simulink model "pendcart"  (Simulink 8.9)
settings: Solver=ode45  StartTime=0.0  StopTime=tsim  RelTol=1e-3  EnableMultiTasking=on
values from neighbouring files (symbols this model uses):
  b = 0.01    [pendcartsim.m]
  c = 0.05    [pendcartsim.m]
  g = 9.82    [pendcartsim.m]
  K1 = -119.0071    [pendcartsim.m]
  K2 = 0.0402    [pendcartsim.m]
  l = 0.5    [pendcartsim.m]
  M = 1    [pendcartsim.m]
  m = 0.5    [pendcartsim.m]
  p = 5.4277    [pendcartsim.m]
  p1 = 25.4277    [pendcartsim.m]
  theta0 = 5*pi/180    (= 0.0872664625997)    [pendcartsim.m]
  Wheel_Radius = 0.035    [pendcartsim.m]
undefined symbols (not defined in the file or in its folder): DiscIntNeverNeededParam, sigbuilder_block, Ts
libraries: powerlib x7
settings Model: Creator=Chris  LastModifiedBy=Administrator
settings OptimizationCC: ExpressionDepthLimit=2147483647  InitFltsAndDblsToZero=on
settings DebuggingCC: AlgebraicLoopMsg=none  SaveWithParameterizedLinksMsg=none
settings GRTTargetCC: TargetFcnLib=ansi_tfl_tmw.mat

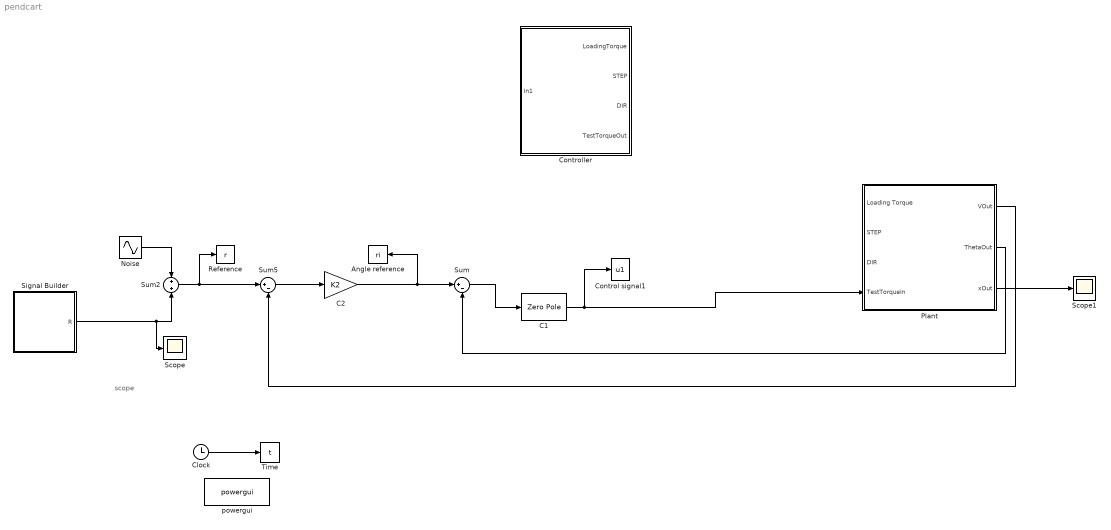
== system pendcart ==
  note: scope
  Angle reference : ToWorkspace  VariableName=ri  SampleTime=-1
  C1 : ZeroPole  Zeros=[-p]  Poles=[-p1]  Gain=[K1]
  C2 : Gain  Gain=K2
  Clock : Clock
  Control signal1 : ToWorkspace  VariableName=u1  SampleTime=-1
  Controller : Subsystem
  "Noise " : Sin  Amplitude=0.01  Frequency=3  SampleTime=0
  Plant : Subsystem
  Reference : ToWorkspace  VariableName=r  SampleTime=-1
  Scope : Scope
  Scope1 : Scope
  Signal Builder : Subsystem  Tag=STV Subsys  LoadFcn=sigbuilder_block('load',[5.5 23 949 425 ]);  StartFcn=sigbuilder_block('start');  StopFcn=sigbuilder_block('stop');  ClipboardFcn=sigbuilder_block('clipboard');  mask(Sigbuilder block){tuvar=[0:10]}
      mask help: Sigbuilder GUI
      mask init:
      | if ~strcmp(get_param(bdroot(gcbh),'SimulationStatus'),'stopped') tuvar = sigbuilder_block('maskInit'); end
      settings: CopyFcn=sigbuilder_block('copy');  DeleteFcn=sigbuilder_block('delete');  ModelCloseFcn=sigbuilder_block('modelClose');  PreSaveFcn=sigbuilder_block('preSave');  PauseFcn=sigbuilder_block('pause')  ContinueFcn=sigbuilder_block('continue')  NameChangeFcn=sigbuilder_block('namechange');  OpenFcn=sigbuilder_block('open',[5.5 23 949 425 ]);  CloseFcn=sigbuilder_block('close');
      mask Display: plot(0, 0, 100, 100,[2, 2, 32, 32, 2], [68, 8, 8, 68, 68],[32, 2], [38, 38], [32, 19, 2],[53, 60, 44], [32, 17, 17, 2],[16, 16, 31, 31]);txt = getActiveGroup(gcbh);text(2, 100, txt,'verticalAlignment', 'top');
  Sum : Sum  Inputs=|+-
  Sum2 : Sum
  Sum5 : Sum  Inputs=|+-
  Time : ToWorkspace  VariableName=t  SampleTime=-1
  powergui : powerlib/powergui  SimulationMode=Discrete  SampleTime=Ts  frequency=60  Iterations=50  frequencyindice=0  Pbase=100e6  ErrMax=1e-4  UnitsV=kV  UnitsW=MW  buscounter=0  FunctionMessages=off  echomessages=off  EnableUseOfTLC=off  CurrentSourceSwitches=off  DisableSnubberDevices=off  DisableRonSwitches=off  DisableVfSwitches=off  DisplayEquations=off  SolverType=Tustin/Backward Euler (TBE)  Interpol=off  ExternalGateDelay=off  methode=off  Ts=0  x0status=blocks  SPID=off  SwTol=0  HookPort=off  RestoreLinks=warning  ResistiveCurrentMeasurement=off  Frange=[0:2:500]  Ylog=off  Xlog=on  ShowGrid=off  save=off  variable=ZData  structure=0  ZoomFFT=on  StartTime=0.0  cycles=1  DisplayStyle=1  fundamental=60  FreqAxis=off  MaxFrequency=1000  frequencyindicesteady=1  RmsSteady=1  display=off
  wires:
  Clock/1 -> Time/1
  Sum5/1 -> C2/1
  C2/1 -> Angle reference/1, Sum/1
  Sum2/1 -> Sum5/1, Reference/1
  "Noise "/1 -> Sum2/1
  Plant/1(VOut) -> Sum5/2
  Plant/2(ThetaOut) -> Sum/2
  ? -> Plant/3(DIR)
  ? -> Plant/2(STEP)
  ? -> Plant/1(Loading Torque)
  C1/1 -> Control signal1/1, Plant/4(TestTorqueIn)
  Sum/1 -> C1/1
  Signal Builder/1(R) -> Scope/1, Sum2/2
  Plant/3(xOut) -> Scope1/1

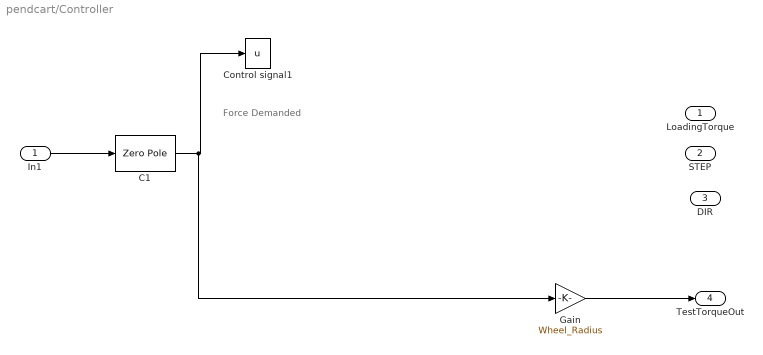
== system pendcart/Controller ==
  note: Force Demanded
  In1 : Inport
  C1 : ZeroPole  Zeros=[-p]  Poles=[-p1]  Gain=[K1]
  Control signal1 : ToWorkspace  VariableName=u  SampleTime=-1
  Gain : Gain  Gain=Wheel_Radius
  LoadingTorque : Outport
  STEP : Outport  Port=2
  DIR : Outport  Port=3
  TestTorqueOut : Outport  Port=4
  wires:
  C1/1 -> Gain/1, Control signal1/1
  In1/1 -> C1/1
  Gain/1 -> TestTorqueOut/1

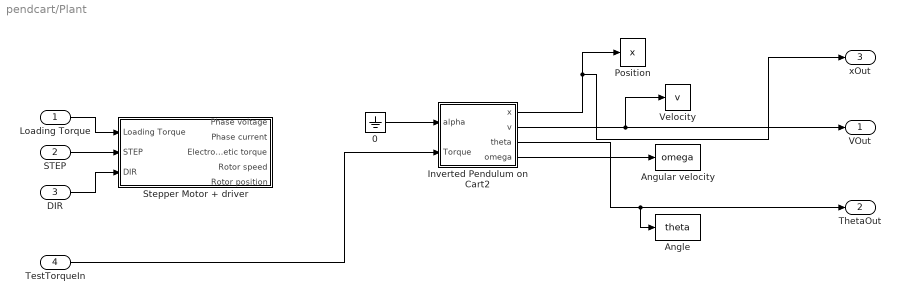
== system pendcart/Plant ==
  Loading Torque : Inport
  STEP : Inport  Port=2
  DIR : Inport  Port=3
  TestTorqueIn : Inport  Port=4
  0 : Ground
  Angle : ToWorkspace  VariableName=theta  SampleTime=-1
  Angular velocity : ToWorkspace  VariableName=omega  SampleTime=-1
  Inverted Pendulum on Cart2 : Subsystem
  Position : ToWorkspace  VariableName=x  SampleTime=-1
  Stepper Motor + driver : Subsystem
  Velocity : ToWorkspace  VariableName=v  SampleTime=-1
  VOut : Outport
  ThetaOut : Outport  Port=2
  xOut : Outport  Port=3
  wires:
  DIR/1 -> Stepper Motor + driver/3(DIR)
  Loading Torque/1 -> Stepper Motor + driver/1(Loading Torque)
  STEP/1 -> Stepper Motor + driver/2(STEP)
  Inverted Pendulum on Cart2/4(omega) -> Angular velocity/1
  Inverted Pendulum on Cart2/1(x) -> xOut/1, Position/1
  Inverted Pendulum on Cart2/3(theta) -> ThetaOut/1, Angle/1
  Inverted Pendulum on Cart2/2(v) -> VOut/1, Velocity/1
  0/1 -> Inverted Pendulum on Cart2/1(alpha)
  TestTorqueIn/1 -> Inverted Pendulum on Cart2/2(Torque)

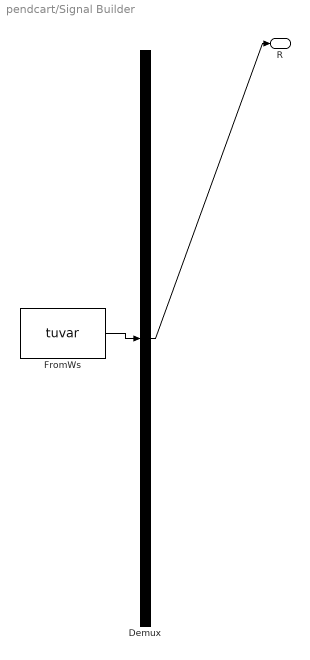
== system pendcart/Signal Builder ==
  Demux : Demux  Tag=STV Demux  Outputs=1
  FromWs : FromWorkspace  Tag=STV FromWs  VariableName=tuvar  SampleTime=0  SigBuilderData=DataTag0  VnvData=DataTag1
      SigBuilderData=|
      | common.afterFinalStr = 'Extrapolate'
      | common.sampleTime = 0
      | dataSet.timeRange = [0 20]
      | dataSet.name = 'Group 1'
      | sbobj.Groups.Name = 'Group 1'
      | sbobj.Groups.Signals.Name = 'R'
      | sbobj.Groups.Signals.XData = [0 8 8 12 12 20]
      | sbobj.Groups.Signals.YData = [0 0.77 1 1 0 0]
      | sbobj.Groups.TimeRange = [0 20]
  R : Outport  Tag=STV Outport
  wires:
  FromWs/1 -> Demux/1
  Demux/1 -> R/1

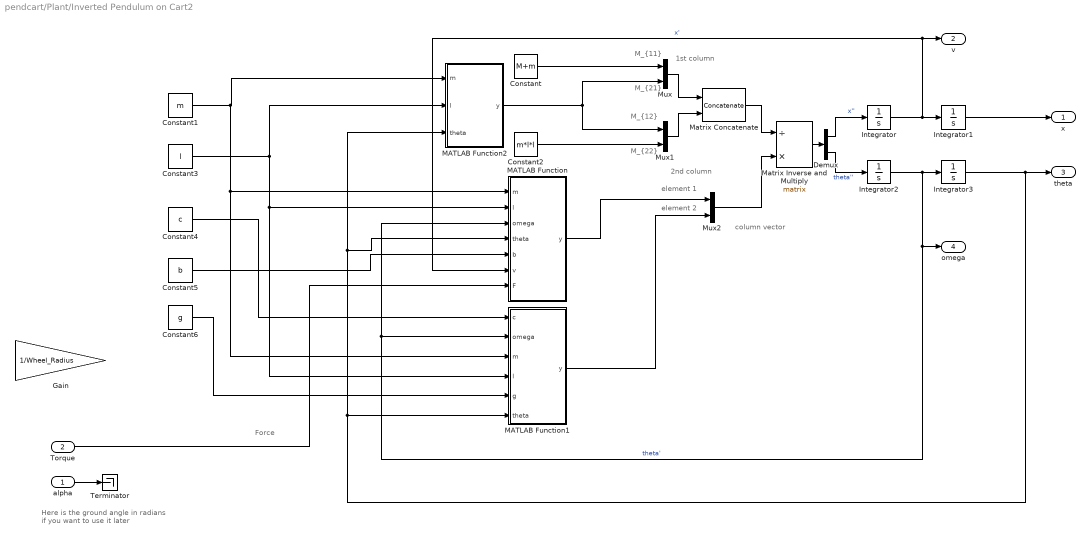
== system pendcart/Plant/Inverted Pendulum on Cart2 ==
  note: Force
  note: 2nd column
  note: M_{21}
  note: 1st column
  note: M_{12}
  note: element 2
  note: Here is the ground angle in
      | radians if you want to use it later
  note: column vector
  note: M_{11}
  note: M_{22}
  note: element 1
  alpha : Inport
  Torque : Inport  Port=2
  Constant : Constant  Value=M+m
  Constant1 : Constant  Value=m
  Constant2 : Constant  Value=m*l*l
  Constant3 : Constant  Value=l
  Constant4 : Constant  Value=c
  Constant5 : Constant  Value=b
  Constant6 : Constant  Value=g
  Demux : Demux  Outputs=2
  Gain : Gain  Gain=1/Wheel_Radius
  Integrator : Integrator
  Integrator1 : Integrator
  Integrator2 : Integrator
  Integrator3 : Integrator  InitialCondition=theta0
  MATLAB Function : MATLAB Function  TreatAsAtomicUnit=on
  MATLAB Function1 : MATLAB Function  TreatAsAtomicUnit=on
  MATLAB Function2 : MATLAB Function  TreatAsAtomicUnit=on
  Matrix Concatenate : Concatenate  Mode=Multidimensional array  ConcatenateDimension=2
  Matrix Inverse and Multiply : Product  Inputs=/*  Multiplication=Matrix(*)
  Mux : Mux  Inputs=2
  Mux1 : Mux  Inputs=2
  Mux2 : Mux  Inputs=2
  Terminator : Terminator
  x : Outport
  v : Outport  Port=2
  theta : Outport  Port=3
  omega : Outport  Port=4
  wires:
  MATLAB Function1/1(y) -> Mux2/2
  Constant1/1 -> MATLAB Function1/3(m), MATLAB Function/1(m), MATLAB Function2/1(m)
  Constant5/1 -> MATLAB Function/5(b)
  Matrix Inverse and Multiply/1 -> Demux/1
  Constant2/1 -> Mux1/2
  Mux2/1 -> Matrix Inverse and Multiply/2
  MATLAB Function/1(y) -> Mux2/1
  Constant4/1 -> MATLAB Function1/1(c)
  Mux1/1 -> Matrix Concatenate/2
  Constant/1 -> Mux/1
  MATLAB Function2/1(y) -> Mux1/1, Mux/2
  Integrator/1 -> Integrator1/1, v/1, MATLAB Function/6(v)  "x'"
  Matrix Concatenate/1 -> Matrix Inverse and Multiply/1
  Integrator1/1 -> x/1
  Demux/2 -> Integrator2/1  "theta''"
  Integrator3/1 -> MATLAB Function/4(theta), MATLAB Function2/3(theta), MATLAB Function1/6(theta), theta/1
  Constant3/1 -> MATLAB Function1/4(l), MATLAB Function/2(l), MATLAB Function2/2(l)
  Mux/1 -> Matrix Concatenate/1
  Integrator2/1 -> Integrator3/1, MATLAB Function/3(omega), MATLAB Function1/2(omega), omega/1  "theta'"
  Constant6/1 -> MATLAB Function1/5(g)
  alpha/1 -> Terminator/1
  Demux/1 -> Integrator/1  "x''"
  Torque/1 -> MATLAB Function/7(F)

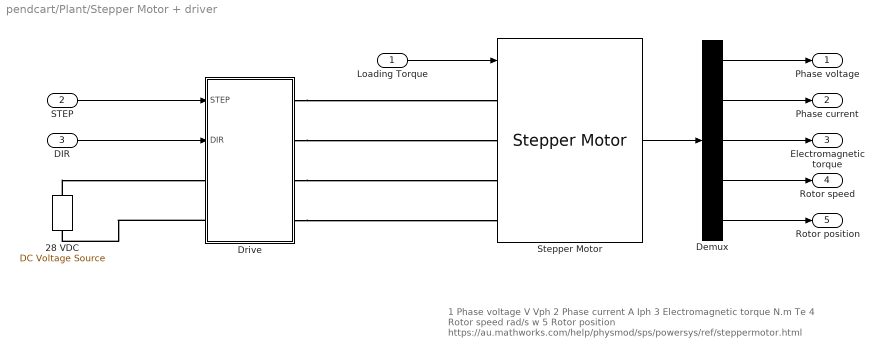
== system pendcart/Plant/Stepper Motor + driver ==
  note: 1
      | Phase voltage
      | V
      | Vph
      |
      | 2
      | Phase current
      | A
      | Iph
      |
      | 3
      | Electromagnetic torque
      | N.m
      | Te
      |
      | 4
      | Rotor speed
      | rad/s
      | w
      |
      | 5
      | Rotor position
      |
      | https://au.mathworks.com/help/physmod/sps/powersys/ref/steppermotor.html
  Loading Torque : Inport
  STEP : Inport  Port=2
  DIR : Inport  Port=3
  28 VDC : powerlib/Electrical Sources/DC Voltage Source  Amplitude=28  Measurements=None
  Demux : Demux  Outputs=5
  Drive : Subsystem  mask{Iref=2, step=500, Ts=Ts}
      mask prompts: Iref "Phase current (A)"; step "Stepping rate (step/s)"; Ts "Sampling time (s)"
      mask init:
      | Nstep=round(1/step/Ts);
  Stepper Motor : powerlib/Machines/Stepper Motor  MotorType=Permanent-magnet / Hybrid  NumberOfPhases_1=2  NumberOfPhases_2=3  PresetModel_1=<empty>  PresetModel_2=<empty>  L=10e-3  Lmax=10e-3  Lmin=2e-3  R=1.2  Step_angle=30  Psim=0.04  Tdm=0.02  J=1e-4/5  B=1e-3  w0=0  pos0=0  TsPowergui=0  TsBlock=-1
      settings: SourceProductName=Simscape Power Systems  SourceProductBaseCode=PS
  Phase voltage : Outport
  Phase current : Outport  Port=2
  Electromagnetic torque : Outport  Port=3
  Rotor speed : Outport  Port=4
  Rotor position : Outport  Port=5
  wires:
  Demux/2 -> Phase current/1
  Loading Torque/1 -> Stepper Motor/1
  Demux/3 -> Electromagnetic torque/1
  Demux/1 -> Phase voltage/1
  Demux/4 -> Rotor speed/1
  Stepper Motor/1 -> Demux/1
  Demux/5 -> Rotor position/1
  DIR/1 -> Drive/2(DIR)
  STEP/1 -> Drive/1(STEP)
  connections:
  Drive/RConn3 -- Stepper Motor/LConn3
  Drive/LConn2 -- 28 VDC/LConn1
  28 VDC/RConn1 -- Drive/LConn1
  Drive/RConn1 -- Stepper Motor/LConn1
  Drive/RConn2 -- Stepper Motor/LConn2
  Drive/RConn4 -- Stepper Motor/LConn4

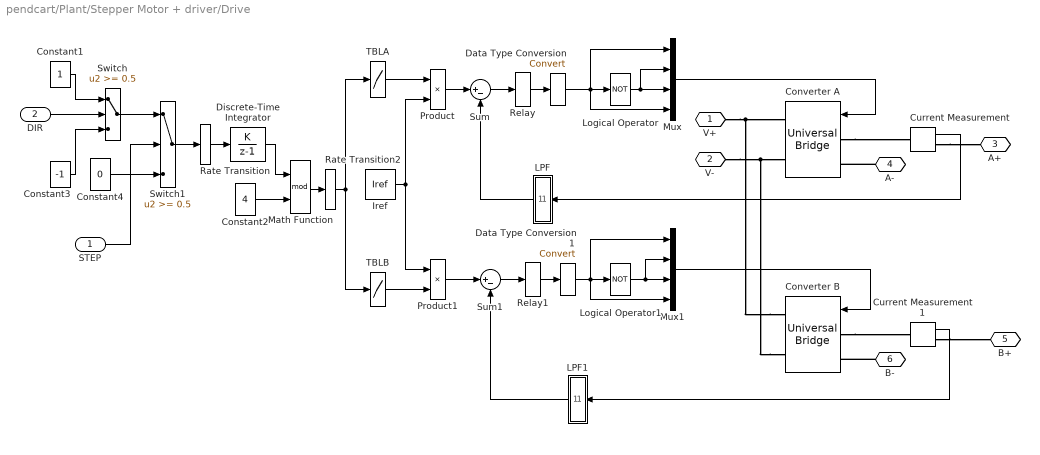
== system pendcart/Plant/Stepper Motor + driver/Drive ==
  STEP : Inport
  DIR : Inport  Port=2
  Constant1 : Constant  SampleTime=Ts
  Constant2 : Constant  Value=4  SampleTime=Nstep*Ts
  Constant3 : Constant  Value=-1  SampleTime=Ts
  Constant4 : Constant  Value=0  SampleTime=Ts
  Converter A : powerlib/Power Electronics/Universal Bridge  Arms=2  SnubberResistance=10000  SnubberCapacitance=inf  Device=MOSFET / Diodes  Ron=1e-3*10  Lon=0  ForwardVoltages="[  0  0  ]"  ForwardVoltage=0  GTOparameters=[ 10e-6 , 20e-6 ]  IGBTparameters=[ 0.5e-6 , 0.5e-6 ]  Measurements=None  Measurements_2=None  converterType=Rectifier
  Converter B : powerlib/Power Electronics/Universal Bridge  Arms=2  SnubberResistance=10000  SnubberCapacitance=inf  Device=MOSFET / Diodes  Ron=1e-3*10  Lon=0  ForwardVoltages="[  0  0  ]"  ForwardVoltage=0  GTOparameters=[ 10e-6 , 20e-6 ]  IGBTparameters=[ 0.5e-6 , 0.5e-6 ]  Measurements=None  Measurements_2=None  converterType=Rectifier
  Current Measurement : powerlib/Measurements/Current Measurement  PhasorSimulation=off  OutputType=Complex  PSBequivalent=0
  Current Measurement1 : powerlib/Measurements/Current Measurement  PhasorSimulation=off  OutputType=Complex  PSBequivalent=0
  Data Type Conversion : DataTypeConversion
  Data Type Conversion1 : DataTypeConversion
  Discrete-Time Integrator : DiscreteIntegrator  IntegratorMethod=Accumulation: Forward Euler  SampleTime=Nstep*Ts  ICPrevOutput=DiscIntNeverNeededParam  ICPrevScaledInput=DiscIntNeverNeededParam
  Iref : Constant  Value=Iref  SampleTime=Ts
  LPF : Subsystem  mask{fc=10000, Ts=Ts}
      mask prompts: fc "Cut-off frequency (Hz)"; Ts "Sampling time (s)"
      mask init:
      | % fa=tf(1,[1/2/pi/fc 1]);
      | % fn=c2d(fa,Ts);
      | % [NN,DD]=tfdata(fn,'v')
      | 
      | NN = [ 0,0.0609];
      | DD = [1.0000,-0.9391];
  LPF1 : Subsystem  mask{fc=10000, Ts=Ts}
      mask prompts: fc "Cut-off frequency (Hz)"; Ts "Sampling time (s)"
      mask init:
      | % fa=tf(1,[1/2/pi/fc 1]);
      | % fn=c2d(fa,Ts);
      | % [NN,DD]=tfdata(fn,'v')
      | 
      | NN = [ 0,0.0609];
      | DD = [1.0000,-0.9391];
  Logical Operator : Logic  Operator=NOT  AllPortsSameDT=off  OutDataTypeStr=boolean
  Logical Operator1 : Logic  Operator=NOT  AllPortsSameDT=off  OutDataTypeStr=boolean
  Math Function : Math  Operator=mod  SampleTime=Nstep*Ts  SaturateOnIntegerOverflow=on
  Mux : Mux
  Mux1 : Mux
  Product : Product  RndMeth=Zero
  Product1 : Product  RndMeth=Zero
  Rate Transition : RateTransition
  Rate Transition2 : RateTransition
  Relay : Relay  OnSwitchValue=0.01  OffSwitchValue=-0.01
  Relay1 : Relay  OnSwitchValue=0.01  OffSwitchValue=-0.01  OutDataTypeStr=Inherit: Inherit via back propagation
  Sum : Sum  Inputs=|+-  OutDataTypeStr=Inherit: Same as first input
  Sum1 : Sum  Inputs=|+-  OutDataTypeStr=Inherit: Same as first input
  Switch : Switch  Threshold=0.5  ZeroCross=off  SampleTime=Ts
  Switch1 : Switch  Threshold=0.5  ZeroCross=off  SampleTime=Ts
  TBLA : Lookup  InputValues=[0:3]  Table=[1 0 -1 0]  SampleTime=Ts
  TBLB : Lookup  InputValues=[0:3]  Table=[0 1 0 -1]  SampleTime=Ts
  V+ : PMIOPort  Port=1  Side=Left
  V- : PMIOPort  Port=2  Side=Left
  A+ : PMIOPort  Port=3  Side=Right
  A- : PMIOPort  Port=4  Side=Right
  B+ : PMIOPort  Port=5  Side=Right
  B- : PMIOPort  Port=6  Side=Right
  wires:
  Constant4/1 -> Switch1/3
  Switch1/1 -> Rate Transition/1
  Switch/1 -> Switch1/1
  STEP/1 -> Switch1/2
  DIR/1 -> Switch/2
  Rate Transition2/1 -> TBLB/1, TBLA/1
  Math Function/1 -> Rate Transition2/1
  Product1/1 -> Sum1/1
  Product/1 -> Sum/1
  Rate Transition/1 -> Discrete-Time Integrator/1
  Constant3/1 -> Switch/3
  Constant1/1 -> Switch/1
  Discrete-Time Integrator/1 -> Math Function/1
  Constant2/1 -> Math Function/2
  Iref/1 -> Product1/1, Product/2
  TBLB/1 -> Product1/2
  TBLA/1 -> Product/1
  LPF1/1(O) -> Sum1/2
  LPF/1(O) -> Sum/2
  Data Type Conversion1/1 -> Mux1/4, Mux1/1, Logical Operator1/1
  Data Type Conversion/1 -> Logical Operator/1, Mux/4, Mux/1
  Current Measurement1/1 -> LPF1/1(I)
  Sum1/1 -> Relay1/1
  Mux1/1 -> Converter B/1
  Logical Operator1/1 -> Mux1/2, Mux1/3
  Relay1/1 -> Data Type Conversion1/1
  Mux/1 -> Converter A/1
  Logical Operator/1 -> Mux/2, Mux/3
  Relay/1 -> Data Type Conversion/1
  Current Measurement/1 -> LPF/1(I)
  Sum/1 -> Relay/1
  connections:
  Converter B/RConn2 -- Converter A/RConn2 -- V-/RConn1
  Converter B/RConn1 -- Converter A/RConn1 -- V+/RConn1
  Current Measurement1/RConn1 -- B+/RConn1
  Converter B/LConn1 -- Current Measurement1/LConn1
  Current Measurement/RConn1 -- A+/RConn1
  Converter A/LConn1 -- Current Measurement/LConn1
  B-/RConn1 -- Converter B/LConn2
  A-/RConn1 -- Converter A/LConn2

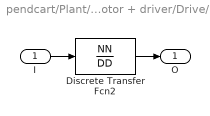
== system pendcart/Plant/Stepper Motor + driver/Drive/LPF ==
  I : Inport
  Discrete Transfer Fcn2 : DiscreteTransferFcn  Numerator=NN  Denominator=DD  SampleTime=Ts
  O : Outport
  wires:
  Discrete Transfer Fcn2/1 -> O/1
  I/1 -> Discrete Transfer Fcn2/1

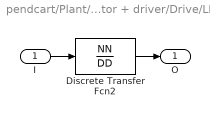
== system pendcart/Plant/Stepper Motor + driver/Drive/LPF1 ==
  I : Inport
  Discrete Transfer Fcn2 : DiscreteTransferFcn  Numerator=NN  Denominator=DD  SampleTime=Ts
  O : Outport
  wires:
  I/1 -> Discrete Transfer Fcn2/1
  Discrete Transfer Fcn2/1 -> O/1

== matlab function Plant/Inverted Pendulum on Cart2/MATLAB Function1 ==
  data: y output double; c input double; omega input double; m input double; l input double; g input double; theta input double
function y  = fcn(c,omega,m,l,g,theta)

y =c*omega+m*l*g*sin(theta);

== matlab function Plant/Inverted Pendulum on Cart2/MATLAB Function ==
  data: y output double; m input double; l input double; omega input double; theta input double; b input double; v input double; F input double
function y = fcn(m,l,omega,theta,b,v,F)

y =m*l*omega*omega*sin(theta)+b*v+F;

== matlab function Plant/Inverted Pendulum on Cart2/MATLAB Function2 ==
  data: y output double; m input double; l input double; theta input double
function y = fcn(m,l,theta)

y =m*l*cos(theta);
